simulink model "dbx_control_v0_02"  (R2015a)
settings: Solver=FixedStepDiscrete  SolverMode=SingleTasking  StartTime=0.0  StopTime=20  FixedStep=T_ctrl  RelTol=1e-3
values from neighbouring files (symbols this model uses):
  A_l_max_x = sqrt( (Max_Thrust*2/m)^2  -  (g*2/3)^2  )    [Run_DBX.m]    (also in simple_all.m = single(A_l_max_x))
  A_M = 2/sqrt(3)*L_M    [SetupComplete.m]    (also in simple_all.m = single(A_M))
  A_z_max = Max_Thrust*3/m    [Run_DBX.m]    (also in simple_all.m = single(A_z_max))
  CG = (m_OE*CG_OE + m_PL*CG_PL)/m    [SetupComplete.m]    (also in simple_all.m = single(CG))
  epsilon = 0.01    [Run_DBX.m]    (also in simple_all.m = single(epsilon))
  Flaps_ang_deg = 0    [FCS_fw_params.m]    (also in simple_all.m = single(Flaps_ang_deg))
  g = 9.81    [SetupComplete.m]    (also in simple_all.m = single(g))
  I_BAC = I_CG + m*[CG(3)^2,0,CG(1)*CG(3);0,CG(1)^2+CG(3)^2,0;CG(1)*CG(3),0,CG(1)^2]    [SetupComplete.m]    (also in simple_all.m = single(I_BAC))
  L_M = 1.20    (= 1.2)    [SetupComplete.m]    (also in simple_all.m = single(L_M))
  m = m_OE + m_PL    (= 14.5)    [SetupComplete.m]    (also in simple_all.m = single(m))
  Roll_pich_sens = single(Roll_pich_sens)    [simple_all.m]
  T_ctrl = 0.01    [Run_DBX.m]    (also in simple_all.m = double(T_ctrl))
  Throtle_sens = single(Throtle_sens)    [simple_all.m]
  v_i0 = sqrt( 1/3*m*g/(2*rho*pi*R^2)  )    [SetupComplete.m]    (also in simple_all.m = single(v_i0))
  Yaw_sens = single(Yaw_sens)    [simple_all.m]
undefined symbols (not defined in the file or in its folder): Hover_eta_23, Hover_throtle_1, Hover_throtle_23, Servo_calib
libraries: DBX_model x29, DBX_Control_lib x15, simulink x8, DBX_Control x3
(part 1 of 2)
settings Model: ExtModeTrigDuration=5000  TunableVars=Flaps_ang_deg,Roll_pich_sens,Throtle_sens,Yaw_sens,p_K_b,p_tau,phi_K_b,phi_f_i,phi_tau,psi_K_b,psi_f_i,psi_tau,q_K_b,q_tau,r_K_b,r_tau,theta_K_b,theta_f_i,theta_tau  TunableVarsStorageClass=Auto,Auto,Auto,Auto,Auto,Auto,Auto,Auto,Auto,Auto,Auto,Auto,Auto,Auto,Auto,Auto,Auto,Auto,Auto  TunableVarsTypeQualifier=,,,,,,,,,,,,,,,,,,  Creator=DavidTorres  LastModifiedBy=David
settings DataIOCC: LimitDataPoints=off  SaveOutput=off  SignalLogging=off  DSMLogging=off  VisualizeSimOutput=off  SaveTime=off
settings OptimizationCC: InlineParams=on  UseDivisionForNetSlopeComputation=on  UseSpecifiedMinMax=on  EfficientFloat2IntCast=on  OptimizeModelRefInitCode=on  MaxStackSize=64  SimCompilerOptimization=on
settings DebuggingCC: SaveWithParameterizedLinksMsg=none  IntegerOverflowMsg=error  StrictBusMsg=ErrorOnBusTreatedAsVector  IntegerSaturationMsg=error
settings HardwareCC: ProdLargestAtomicInteger=Long  ProdLargestAtomicFloat=Double  ProdIntDivRoundTo=Zero  ProdEndianess=LittleEndian  ProdHWDeviceType=Generic->32-bit x86 compatible  TargetLongLongMode=on  TargetIntDivRoundTo=Zero  TargetEndianess=LittleEndian  TargetHWDeviceType=MATLAB Host  ProdEqTarget=off
settings ModelReferenceCC: ModelReferenceNumInstancesAllowed=Single  ModelReferencePassRootInputsByReference=off
settings RTWCC: SystemTargetFile=ert.tlc  GenCodeOnly=on  TemplateMakefile=ert_default_tmf  Description=Embedded Coder  BuildConfiguration=Faster Runs
settings CodeAppCC: IgnoreCustomStorageClasses=off
settings ERTTargetCC: GenerateSampleERTMain=off  ParMdlRefBuildCompliant=on  CompOptLevelCompliant=on  ConcurrentExecutionCompliant=on  ERTFirstTimeCompliant=on  SupportNonFinite=off  SupportComplex=off  SupportContinuousTime=off  ModelStepFunctionPrototypeControlCompliant=on  CPPClassGenCompliant=on  InlinedParameterPlacement=Hierarchical  ERTCustomFileTemplate=example_file_process.tlc

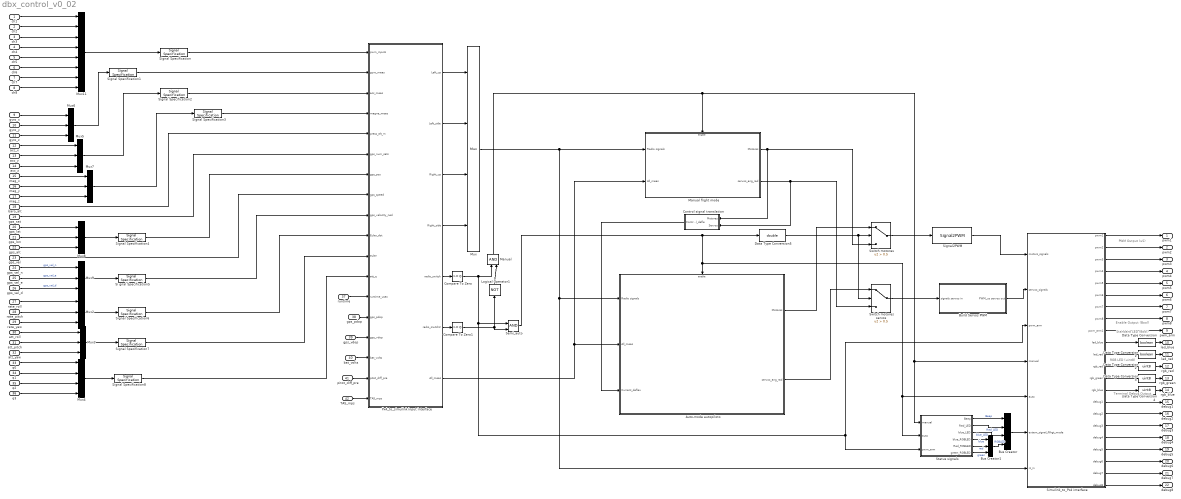
== system dbx_control_v0_02 ==
  note: Terminal Debug Output
  note: RGB LED (uint8)
  note: Standard LED (Bool)
  note: PWM Output (uS)
  note: Enable Output (Bool)
  ch1 : Inport  PortDimensions=[1,1]  SampleTime=T_ctrl
  ch2 : Inport  Port=2  PortDimensions=[1,1]  SampleTime=T_ctrl
  ch3 : Inport  Port=3  PortDimensions=[1,1]  SampleTime=T_ctrl
  ch4 : Inport  Port=4  PortDimensions=[1,1]  SampleTime=T_ctrl
  ch5 : Inport  Port=5  PortDimensions=[1,1]  SampleTime=T_ctrl
  ch6 : Inport  Port=6  PortDimensions=[1,1]  SampleTime=T_ctrl
  ch7 : Inport  Port=7  PortDimensions=[1,1]  SampleTime=T_ctrl
  ch8 : Inport  Port=8  PortDimensions=[1,1]  SampleTime=T_ctrl
  gyro_x : Inport  Port=9  PortDimensions=[1,1]  SampleTime=T_ctrl
  gyro_y : Inport  Port=10  PortDimensions=[1,1]  SampleTime=T_ctrl
  gyro_z : Inport  Port=11  PortDimensions=[1,1]  SampleTime=T_ctrl
  acc_x : Inport  Port=12  PortDimensions=[1,1]  SampleTime=T_ctrl
  acc_y : Inport  Port=13  PortDimensions=[1,1]  SampleTime=T_ctrl
  acc_z : Inport  Port=14  PortDimensions=[1,1]  SampleTime=T_ctrl
  mag_x : Inport  Port=15  PortDimensions=[1,1]  SampleTime=T_ctrl
  mag_y : Inport  Port=16  PortDimensions=[1,1]  SampleTime=T_ctrl
  mag_z : Inport  Port=17  PortDimensions=[1,1]  SampleTime=T_ctrl
  baro_alt : Inport  Port=18  PortDimensions=[1,1]  SampleTime=T_ctrl
  gps_sat : Inport  Port=19  PortDimensions=[1,1]  SampleTime=T_ctrl
  gps_lat : Inport  Port=20  PortDimensions=[1,1]  SampleTime=T_ctrl
  gps_lon : Inport  Port=21  PortDimensions=[1,1]  SampleTime=T_ctrl
  gps_alt : Inport  Port=22  PortDimensions=[1,1]  SampleTime=T_ctrl
  gps_vel : Inport  Port=23  PortDimensions=[1,1]  SampleTime=T_ctrl
  gps_vel_n : Inport  Port=24  PortDimensions=[1,1]  SampleTime=T_ctrl
  gps_vel_e : Inport  Port=25  PortDimensions=[1,1]  SampleTime=T_ctrl
  gps_vel_d : Inport  Port=26  PortDimensions=[1,1]  SampleTime=T_ctrl
  rate_roll : Inport  Port=27  PortDimensions=[1,1]  SampleTime=T_ctrl
  rate_pitch : Inport  Port=28  PortDimensions=[1,1]  SampleTime=T_ctrl
  rate_yaw : Inport  Port=29  PortDimensions=[1,1]  SampleTime=T_ctrl
  att_roll : Inport  Port=30  PortDimensions=[1,1]  SampleTime=T_ctrl
  att_pitch : Inport  Port=31  PortDimensions=[1,1]  SampleTime=T_ctrl
  att_yaw : Inport  Port=32  PortDimensions=[1,1]  SampleTime=T_ctrl
  q0 : Inport  Port=33  PortDimensions=[1,1]  SampleTime=T_ctrl
  q1 : Inport  Port=34  PortDimensions=[1,1]  SampleTime=T_ctrl
  q2 : Inport  Port=35  PortDimensions=[1,1]  SampleTime=T_ctrl
  q3 : Inport  Port=36  PortDimensions=[1,1]  SampleTime=T_ctrl
  runtime : Inport  Port=37  PortDimensions=[1,1]  SampleTime=T_ctrl
  gps_pdop : Inport  Port=38  PortDimensions=[1,1]  SampleTime=T_ctrl
  gps_vdop : Inport  Port=39  PortDimensions=[1,1]  SampleTime=T_ctrl
  bat_volts : Inport  Port=40  PortDimensions=[1,1]  SampleTime=T_ctrl
  pitot_diff_pre : Inport  Port=41  SampleTime=T_ctrl
  TAS_mps : Inport  Port=42  SampleTime=T_ctrl
  Auto-mode autopiloto : Subsystem  TreatAsAtomicUnit=on
  Build Servos PWM : Subsystem  TreatAsAtomicUnit=on
  Bus Creator : BusCreator
  Bus Creator1 : BusCreator  Inputs=3
  Compare To Zero : simulink/Logic and Bit Operations/Compare To Zero  relop=>=  OutDataTypeStr=boolean
  Compare To Zero1 : simulink/Logic and Bit Operations/Compare To Zero  relop=>=  OutDataTypeStr=boolean
  Control signal translation : Subsystem  TreatAsAtomicUnit=on
  Data Type Conversion : DataTypeConversion  OutDataTypeStr=boolean
  Data Type Conversion1 : DataTypeConversion  OutDataTypeStr=boolean
  Data Type Conversion2 : DataTypeConversion  OutDataTypeStr=uint8
  Data Type Conversion3 : DataTypeConversion  OutDataTypeStr=uint8
  Data Type Conversion4 : DataTypeConversion  OutDataTypeStr=uint8
  Data Type Conversion5 : DataTypeConversion  OutDataTypeStr=double
  Logical Operator1 : Logic  Operator=NOT  IconShape=distinctive  AllPortsSameDT=off  OutDataTypeStr=boolean
  Manual : Logic  IconShape=distinctive  AllPortsSameDT=off  OutDataTypeStr=boolean
  Manual flight mode : Subsystem  TreatAsAtomicUnit=on
  Mux : Mux
  Mux11 : Mux  Inputs=8
  Mux{2..3,5..9} (7 alike) : Mux  Inputs=3
  Mux4 : Mux
  Px4_to_simulink input interface : Subsystem
  Semi_auto : Logic  IconShape=distinctive  AllPortsSameDT=off  OutDataTypeStr=boolean
  Si gnal Specification5 : SignalSpecification  Dimensions=[3,1]
  Signal Specification : SignalSpecification  Dimensions=[8,1]
  Signal Specification{1..4,6..7} (6 alike) : SignalSpecification  Dimensions=[3,1]
  Signal Specification8 : SignalSpecification  Dimensions=[4,1]
  Signal2PWM : DBX_model/Signal2PWM  b=1  d=0  a=1900  c=1100
  Simulink_to_Px4 interface : Subsystem
  Status signals : Subsystem  TreatAsAtomicUnit=on
  Switch motores : Switch  Criteria=u2 > Threshold  Threshold=0.5
  Switch motores servos : Switch  Criteria=u2 > Threshold  Threshold=0.5
  pwm1 : Outport  PortDimensions=[1,1]
  pwm2 : Outport  Port=2  PortDimensions=[1,1]
  pwm3 : Outport  Port=3  PortDimensions=[1,1]
  pwm4 : Outport  Port=4  PortDimensions=[1,1]
  pwm5 : Outport  Port=5  PortDimensions=[1,1]
  pwm6 : Outport  Port=6  PortDimensions=[1,1]
  pwm7 : Outport  Port=7  PortDimensions=[1,1]
  pwm8 : Outport  Port=8  PortDimensions=[1,1]
  pwm_arm : Outport  Port=9  PortDimensions=[1,1]
  led_blue : Outport  Port=10  OutDataTypeStr=boolean  PortDimensions=[1,1]
  led_red : Outport  Port=11  OutDataTypeStr=boolean  PortDimensions=[1,1]
  rgb_red : Outport  Port=12  OutDataTypeStr=uint8  PortDimensions=[1,1]
  rgb_green : Outport  Port=13  OutDataTypeStr=uint8  PortDimensions=[1,1]
  rgb_blue : Outport  Port=14  OutDataTypeStr=uint8  PortDimensions=[1,1]
  debug1 : Outport  Port=15  PortDimensions=[1,1]
  debug2 : Outport  Port=16  PortDimensions=[1,1]
  debug3 : Outport  Port=17  PortDimensions=[1,1]
  debug4 : Outport  Port=18  PortDimensions=[1,1]
  debug5 : Outport  Port=19  PortDimensions=[1,1]
  debug6 : Outport  Port=20  PortDimensions=[1,1]
  debug7 : Outport  Port=21  PortDimensions=[1,1]
  debug8 : Outport  Port=22  PortDimensions=[1,1]
  wires:
  Switch motores/1 -> Signal2PWM/1
  Switch motores servos/1 -> Build Servos PWM/1(signals servos in)
  Status signals/1(Beep) -> Bus Creator/1  "Beep"
  Status signals/2(Red_LED) -> Bus Creator/2  "Red_LED"
  Status signals/3(blue_LED) -> Bus Creator/3  "blue_LED"
  Status signals/4(blue_RGBLED) -> Bus Creator1/1  "blue"
  Status signals/5(Red_RGBLED) -> Bus Creator1/2  "red"
  Status signals/6(green_RGBLED) -> Bus Creator1/3  "green"
  Bus Creator1/1 -> Bus Creator/4  "RGBLED"
  Simulink_to_Px4 interface/1(pwm1) -> pwm1/1
  Simulink_to_Px4 interface/2(pwm2) -> pwm2/1
  Simulink_to_Px4 interface/3(pwm3) -> pwm3/1
  Simulink_to_Px4 interface/4(pwm4) -> pwm4/1
  Simulink_to_Px4 interface/5(pwm5) -> pwm5/1
  Simulink_to_Px4 interface/6(pwm6) -> pwm6/1
  Simulink_to_Px4 interface/7(pwm7) -> pwm7/1
  Simulink_to_Px4 interface/8(pwm8) -> pwm8/1
  Simulink_to_Px4 interface/10(led_blue) -> Data Type Conversion/1
  Simulink_to_Px4 interface/11(led_red) -> Data Type Conversion1/1
  Simulink_to_Px4 interface/15(debug1) -> debug1/1
  Simulink_to_Px4 interface/17(debug3) -> debug3/1
  Simulink_to_Px4 interface/18(debug4) -> debug4/1
  Simulink_to_Px4 interface/9(pwm_arm1) -> pwm_arm/1
  Simulink_to_Px4 interface/12(rgb_red) -> Data Type Conversion2/1
  Simulink_to_Px4 interface/13(rgb_green) -> Data Type Conversion3/1
  Simulink_to_Px4 interface/14(rgb_blue) -> Data Type Conversion4/1
  Simulink_to_Px4 interface/20(debug6) -> debug6/1
  Simulink_to_Px4 interface/21(debug7) -> debug7/1
  Simulink_to_Px4 interface/22(debug8) -> debug8/1
  Simulink_to_Px4 interface/19(debug5) -> debug5/1
  Data Type Conversion/1 -> led_blue/1
  Data Type Conversion1/1 -> led_red/1
  Data Type Conversion2/1 -> rgb_red/1
  Data Type Conversion3/1 -> rgb_green/1
  Data Type Conversion4/1 -> rgb_blue/1
  Simulink_to_Px4 interface/16(debug2) -> debug2/1
  Signal2PWM/1 -> Simulink_to_Px4 interface/1(motors_signals)
  Build Servos PWM/1(PWM_us servos out) -> Simulink_to_Px4 interface/2(servos_signals)
  Bus Creator/1 -> Simulink_to_Px4 interface/6(extern_signal_flihgt_mode)
  baro_alt/1 -> Px4_to_simulink input interface/5(press_alt_m)
  gyro_z/1 -> Mux6/3
  gyro_y/1 -> Mux6/2
  gyro_x/1 -> Mux6/1
  acc_z/1 -> Mux5/3
  acc_y/1 -> Mux5/2
  acc_x/1 -> Mux5/1
  mag_x/1 -> Mux7/1
  mag_y/1 -> Mux7/2
  mag_z/1 -> Mux7/3
  ch1/1 -> Mux11/1
  ch2/1 -> Mux11/2
  ch3/1 -> Mux11/3
  ch4/1 -> Mux11/4
  ch5/1 -> Mux11/5
  ch6/1 -> Mux11/6
  runtime/1 -> Px4_to_simulink input interface/13(runtime_usec)
  ch7/1 -> Mux11/7
  ch8/1 -> Mux11/8
  att_roll/1 -> Mux3/1
  att_pitch/1 -> Mux3/2
  att_yaw/1 -> Mux3/3
  q0/1 -> Mux4/1
  q1/1 -> Mux4/2
  q2/1 -> Mux4/3
  q3/1 -> Mux4/4
  rate_roll/1 -> Mux2/1
  rate_pitch/1 -> Mux2/2
  rate_yaw/1 -> Mux2/3
  gps_vel_n/1 -> Mux9/1  "gps_vel_n"
  gps_vel_e/1 -> Mux9/2  "gps_vel_e"
  gps_vel_d/1 -> Mux9/3  "gps_vel_d"
  gps_lat/1 -> Mux8/1
  gps_lon/1 -> Mux8/2
  gps_alt/1 -> Mux8/3
  gps_vel/1 -> Px4_to_simulink input interface/8(gps_speed)
  gps_sat/1 -> Px4_to_simulink input interface/6(gps_num_sats)
  Mux2/1 -> Signal Specification6/1
  Mux3/1 -> Signal Specification7/1
  Mux4/1 -> Signal Specification8/1
  Mux5/1 -> Signal Specification2/1
  Mux6/1 -> Signal Specification1/1
  Mux8/1 -> Signal Specification4/1
  Mux7/1 -> Signal Specification3/1
  Mux11/1 -> Signal Specification/1
  Mux9/1 -> Si gnal Specification5/1
  gps_pdop/1 -> Px4_to_simulink input interface/14(gps_pdop)
  gps_vdop/1 -> Px4_to_simulink input interface/15(gps_vdop)
  bat_volts/1 -> Px4_to_simulink input interface/16(bat_volts)
  Signal Specification/1 -> Px4_to_simulink input interface/1(pwm_inputs)
  Signal Specification1/1 -> Px4_to_simulink input interface/2(gyro_meas)
  Signal Specification2/1 -> Px4_to_simulink input interface/3(acc_meas)
  Signal Specification3/1 -> Px4_to_simulink input interface/4(magne_meas)
  Signal Specification4/1 -> Px4_to_simulink input interface/7(gps_pos)
  Si gnal Specification5/1 -> Px4_to_simulink input interface/9(gps_velocity_ned)
  Signal Specification6/1 -> Px4_to_simulink input interface/10(Euler_dot)
  Signal Specification7/1 -> Px4_to_simulink input interface/11(euler)
  Signal Specification8/1 -> Px4_to_simulink input interface/12(att_q)
  pitot_diff_pre/1 -> Px4_to_simulink input interface/17(pitot_diff_pre)
  Px4_to_simulink input interface/5(radio_switch) -> Compare To Zero/1
  Px4_to_simulink input interface/6(radio_siwtch2) -> Compare To Zero1/1
  Compare To Zero/1 -> Semi_auto/1, Simulink_to_Px4 interface/3(pwm_arm), Status signals/3(pwm_arm), Manual/1
  Compare To Zero1/1 -> Logical Operator1/1, Semi_auto/2
  Manual/1 -> Simulink_to_Px4 interface/4(manual), Status signals/1(manual), Manual flight mode/Enable
  Manual flight mode/2(servos_ang_rad) -> Control signal translation/2(Servos), Switch motores servos/3
  Auto-mode autopiloto/1(Motores) -> Switch motores/1
  Auto-mode autopiloto/2(servos_ang_rad) -> Switch motores servos/1
  Semi_auto/1 -> Data Type Conversion5/1, Simulink_to_Px4 interface/5(auto), Status signals/2(auto), Auto-mode autopiloto/Enable
  Data Type Conversion5/1 -> Switch motores servos/2, Switch motores/2
  Px4_to_simulink input interface/4(Right_side) -> Mux/4
  Px4_to_simulink input interface/3(Right_up) -> Mux/3
  Px4_to_simulink input interface/2(Left_side) -> Mux/2
  Px4_to_simulink input interface/1(Left_up) -> Mux/1
  Px4_to_simulink input interface/7(All_meas) -> Manual flight mode/2(All_meas), Auto-mode autopiloto/2(All_meas)
  Mux/1 -> Manual flight mode/1(Radio signals), Simulink_to_Px4 interface/7(rc_in), Auto-mode autopiloto/1(Radio signals)
  TAS_mps/1 -> Px4_to_simulink input interface/18(TAS_mps)
  Logical Operator1/1 -> Manual/2
  Manual flight mode/1(Motores) -> Switch motores/3, Control signal translation/1(Motores)
  Control signal translation/1(Control_defle) -> Auto-mode autopiloto/3(Current_deflex)

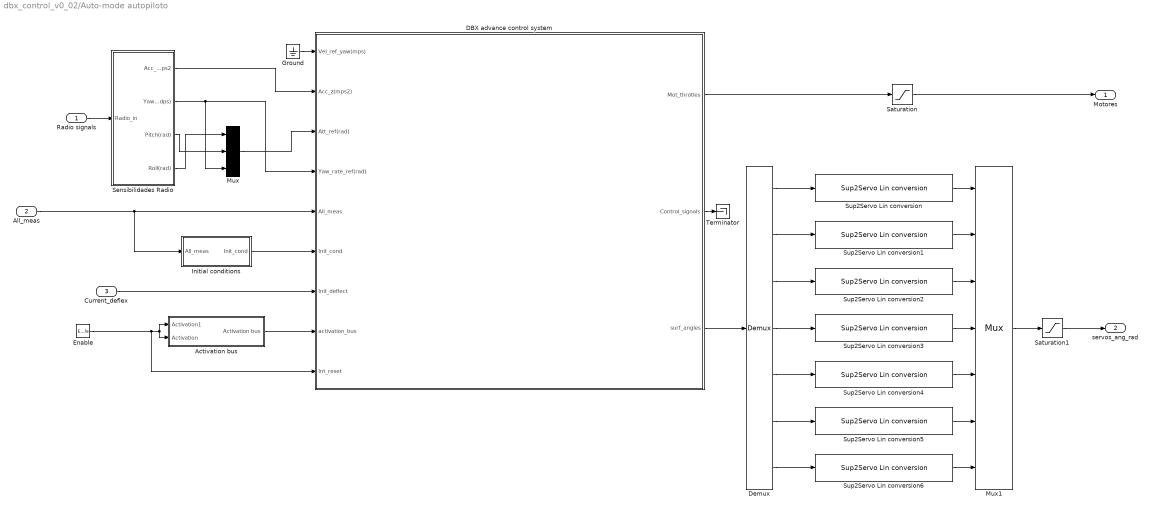
== system dbx_control_v0_02/Auto-mode autopiloto ==
  Radio signals : Inport
  All_meas : Inport  Port=2
  Current_deflex : Inport  Port=3
  Enable : EnablePort  ShowOutputPort=on
  Activation bus : Subsystem  TreatAsAtomicUnit=on
  DBX advance control system : Subsystem
  Demux : Demux  Outputs=7
  "Ground " : Ground
  Initial conditions : Subsystem  TreatAsAtomicUnit=on
  Mux : Mux  Inputs=3
  Mux1 : Mux  Inputs=7
  Saturation : Saturate  UpperLimit=1  LowerLimit=0
  Saturation1 : Saturate  UpperLimit=deg2rad(90)  LowerLimit=-deg2rad(90)
  Sensibilidades Radio : Subsystem  TreatAsAtomicUnit=on
  Sup2Servo Lin conversion : DBX_model/Sup2Servo Lin conversion  Gain=Servo_calib.Servo1.Pendiente_Sup_Servo  Bias=Servo_calib.Servo1.Sup_rad_0
  Sup2Servo Lin conversion1 : DBX_model/Sup2Servo Lin conversion  Gain=Servo_calib.Servo2.Pendiente_Sup_Servo  Bias=Servo_calib.Servo2.Sup_rad_0
  Sup2Servo Lin conversion2 : DBX_model/Sup2Servo Lin conversion  Gain=Servo_calib.Servo3.Pendiente_Sup_Servo  Bias=Servo_calib.Servo3.Sup_rad_0
  Sup2Servo Lin conversion3 : DBX_model/Sup2Servo Lin conversion  Gain=Servo_calib.Servo4.Pendiente_Sup_Servo  Bias=Servo_calib.Servo4.Sup_rad_0
  Sup2Servo Lin conversion4 : DBX_model/Sup2Servo Lin conversion  Gain=Servo_calib.Servo5.Pendiente_Sup_Servo  Bias=Servo_calib.Servo5.Sup_rad_0
  Sup2Servo Lin conversion5 : DBX_model/Sup2Servo Lin conversion  Gain=Servo_calib.Servo6.Pendiente_Sup_Servo  Bias=Servo_calib.Servo6.Sup_rad_0
  Sup2Servo Lin conversion6 : DBX_model/Sup2Servo Lin conversion  Gain=Servo_calib.Servo7.Pendiente_Sup_Servo  Bias=Servo_calib.Servo7.Sup_rad_0
  Terminator : Terminator
  Motores : Outport
  servos_ang_rad : Outport  Port=2
  wires:
  DBX advance control system/1(Mot_throtles) -> Saturation/1
  Saturation/1 -> Motores/1
  Mux1/1 -> Saturation1/1
  Saturation1/1 -> servos_ang_rad/1
  Sup2Servo Lin conversion/1 -> Mux1/1
  Sup2Servo Lin conversion1/1 -> Mux1/2
  Sup2Servo Lin conversion2/1 -> Mux1/3
  Sup2Servo Lin conversion3/1 -> Mux1/4
  Sup2Servo Lin conversion4/1 -> Mux1/5
  Sup2Servo Lin conversion5/1 -> Mux1/6
  Sup2Servo Lin conversion6/1 -> Mux1/7
  All_meas/1 -> Initial conditions/1(All_meas), DBX advance control system/5(All_meas)
  DBX advance control system/3(surf_angles) -> Demux/1
  Demux/1 -> Sup2Servo Lin conversion/1
  Demux/2 -> Sup2Servo Lin conversion1/1
  Demux/3 -> Sup2Servo Lin conversion2/1
  Demux/4 -> Sup2Servo Lin conversion3/1
  Demux/5 -> Sup2Servo Lin conversion4/1
  Demux/6 -> Sup2Servo Lin conversion5/1
  Demux/7 -> Sup2Servo Lin conversion6/1
  Radio signals/1 -> Sensibilidades Radio/1(Radio_in)
  Sensibilidades Radio/1(Acc_z_mps2) -> DBX advance control system/2(Acc_z(mps2))
  Mux/1 -> DBX advance control system/3(Att_ref(rad))
  "Ground "/1 -> DBX advance control system/1(Vel_ref_yaw(mps))
  Sensibilidades Radio/2(Yaw(radps)) -> Mux/3, DBX advance control system/4(Yaw_rate_ref(rad))
  Sensibilidades Radio/4(Roll(rad)) -> Mux/1
  Sensibilidades Radio/3(Pitch(rad)) -> Mux/2
  Activation bus/1(Activation bus) -> DBX advance control system/8(activation_bus)
  Enable/1 -> DBX advance control system/9(Int_reset), Activation bus/2(Activation), Activation bus/1(Activation1)
  Initial conditions/1(Init_cond) -> DBX advance control system/6(Init_cond)
  Current_deflex/1 -> DBX advance control system/7(Init_deflect)
  DBX advance control system/2(Control_signals) -> Terminator/1

== system dbx_control_v0_02/Build Servos PWM ==
  note: Estos 4 ultimos significa que
      | los ejes de los servos deben
      | apuntar el la direccion +y
  note: Control input
      | Rango
      | Direccion rot/Dir servos
      | Rango del servo
      |
      | eta_1 (rad) (Pan arm 1)
      | -90,90
      | -1
      | 180
      |
      | eta_2 (rad) (Pan arm 2
      | -90,90
      | -1
      | 180
      |
      | eta_3 (rad) (Pan arm 3)
      | -90,90
      | 1
      | 180
      |
      | Rudervator Left (rad)
      | -90,90
      | 1
      | 180
      |
      | Rudervator Right (rad)
      | -90,90
      | 1
      | 180
      |
      | Aileron Left (rad)
      | -90,90
      | 1
      | 180
      |
      | Aielron Right (rad)
      | -90,90
      | 1
      | 180
  signals servos in : Inport
  Demux : Demux  Outputs=7
  Mux : Mux  Inputs=7
  Signal2PWM{,1..6} (7 alike) : DBX_model/Signal2PWM  b=deg2rad(90)  d=-deg2rad(90)  a=1900  c=1100
  PWM_us servos out : Outport
  wires:
  Mux/1 -> PWM_us servos out/1
  signals servos in/1 -> Demux/1
  Demux/6 -> Signal2PWM5/1
  Demux/5 -> Signal2PWM4/1
  Demux/4 -> Signal2PWM3/1
  Demux/3 -> Signal2PWM2/1
  Demux/2 -> Signal2PWM1/1
  Demux/1 -> Signal2PWM/1
  Signal2PWM/1 -> Mux/1
  Signal2PWM1/1 -> Mux/2
  Signal2PWM3/1 -> Mux/4
  Signal2PWM4/1 -> Mux/5
  Signal2PWM2/1 -> Mux/3
  Signal2PWM5/1 -> Mux/6
  Demux/7 -> Signal2PWM6/1
  Signal2PWM6/1 -> Mux/7

== system dbx_control_v0_02/Control signal translation ==
  Motores : Inport
  Servos : Inport  Port=2
  Demux : Demux  Outputs=3
  Ground{,1..4} (5 alike) : Ground
  Mux1 : Mux  Inputs=9
  Selector : Selector  InputPortWidth=7  Indices=3
  Servo2Sup Lin conversion : DBX_model/Servo2Sup Lin conversion  Gain=Servo_calib.Servo3.Pendiente_Sup_Servo  Bias=Servo_calib.Servo3.Sup_rad_0
  Control_defle : Outport
  wires:
  Mux1/1 -> Control_defle/1
  Demux/1 -> Mux1/1
  Servos/1 -> Selector/1
  Demux/2 -> Mux1/3
  Demux/3 -> Mux1/5
  Ground/1 -> Mux1/2
  Ground1/1 -> Mux1/4
  Ground2/1 -> Mux1/7
  Ground3/1 -> Mux1/8
  Ground4/1 -> Mux1/9
  Servo2Sup Lin conversion/1 -> Mux1/6
  Motores/1 -> Demux/1
  Selector/1 -> Servo2Sup Lin conversion/1

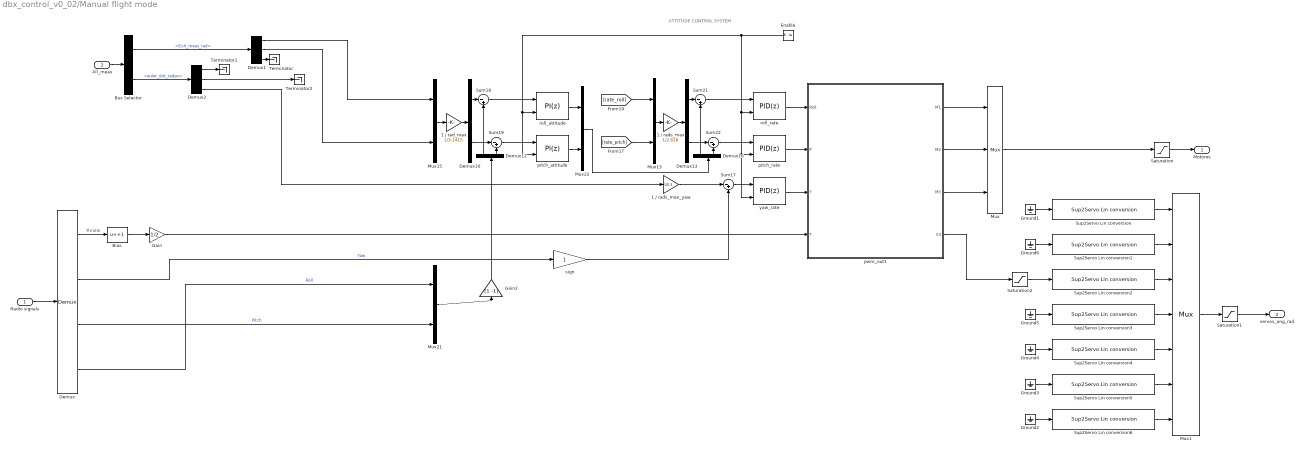
== system dbx_control_v0_02/Manual flight mode ==
  note: ATTITUDE CONTROL SYSTEM
  Radio signals : Inport
  All_meas : Inport  Port=2
  Enable : EnablePort  ShowOutputPort=on
  1 / rad_max : Gain  Gain=1/3.1415
  1 / rads_max : Gain  Gain=1/2.618
  1 / rads_max_yaw : Gain  Gain=1/5.3
  Bias : Bias  Bias=+1
  Bus Selector : BusSelector  OutputSignals=Meas.Eulr_meas_rad,Meas.euler_dot_radps
  Demux : Demux
  Demux1 : Demux  Outputs=3
  Demux{10,12..13,16} (4 alike) : Demux  Outputs=2
  Demux2 : Demux  Outputs=3
  Gain : Gain  Gain=1/2
  Gain2 : Gain  Gain=[1 -1]
  Ground{1..6} (6 alike) : Ground
  Mux : Mux  Inputs=3
  Mux1 : Mux  Inputs=7
  Mux{13,15,21..22} (4 alike) : Mux  Inputs=2
  Saturation : Saturate  UpperLimit=1  LowerLimit=0
  Saturation1 : Saturate  UpperLimit=deg2rad(90)  LowerLimit=-deg2rad(90)
  Saturation2 : Saturate  UpperLimit=deg2rad(20)  LowerLimit=-deg2rad(20)
  Sum{17..19,21..22} (5 alike) : Sum  Inputs=|-+
  Sup2Servo Lin conversion : DBX_model/Sup2Servo Lin conversion  Gain=Servo_calib.Servo1.Pendiente_Sup_Servo  Bias=Servo_calib.Servo1.Sup_rad_0
  Sup2Servo Lin conversion1 : DBX_model/Sup2Servo Lin conversion  Gain=Servo_calib.Servo2.Pendiente_Sup_Servo  Bias=Servo_calib.Servo2.Sup_rad_0
  Sup2Servo Lin conversion2 : DBX_model/Sup2Servo Lin conversion  Gain=Servo_calib.Servo3.Pendiente_Sup_Servo  Bias=Servo_calib.Servo3.Sup_rad_0
  Sup2Servo Lin conversion3 : DBX_model/Sup2Servo Lin conversion  Gain=Servo_calib.Servo4.Pendiente_Sup_Servo  Bias=Servo_calib.Servo4.Sup_rad_0
  Sup2Servo Lin conversion4 : DBX_model/Sup2Servo Lin conversion  Gain=Servo_calib.Servo5.Pendiente_Sup_Servo  Bias=Servo_calib.Servo5.Sup_rad_0
  Sup2Servo Lin conversion5 : DBX_model/Sup2Servo Lin conversion  Gain=Servo_calib.Servo6.Pendiente_Sup_Servo  Bias=Servo_calib.Servo6.Sup_rad_0
  Sup2Servo Lin conversion6 : DBX_model/Sup2Servo Lin conversion  Gain=Servo_calib.Servo7.Pendiente_Sup_Servo  Bias=Servo_calib.Servo7.Sup_rad_0
  Terminator : Terminator
  Terminator1 : Terminator
  Terminator2 : Terminator
  pitch_attitude : simulink/Continuous/PID Controller  Controller=PI  TimeDomain=Discrete-time  SampleTime=-1  IntegratorMethod=Forward Euler  FilterMethod=Forward Euler  Form=Parallel  UseFilter=on  ControllerParametersSource=internal  P=0.4  I=0.1  D=0  N=100  InitialConditionSource=internal  InitialConditionForIntegrator=0  InitialConditionForFilter=0  ExternalReset=either  LimitOutput=on  UpperSaturationLimit=1  LowerSaturationLimit=-1  LinearizeAsGain=on  AntiWindupMode=none  Kb=1  TrackingMode=off  Kt=1  PParamMin=[]  PParamMax=[]  IParamMin=[]  IParamMax=[]  DParamMin=[]  DParamMax=[]  NParamMin=[]  NParamMax=[]  KbParamMin=[]  KbParamMax=[]  KtParamMin=[]  KtParamMax=[]  POutMin=[]  POutMax=[]  IOutMin=[]  IOutMax=[]  DOutMin=[]  DOutMax=[]  NOutMin=[]  NOutMax=[]  KbOutMin=[]  KbOutMax=[]  KtOutMin=[]  KtOutMax=[]  IntegratorOutMin=[]  IntegratorOutMax=[]  FilterOutMin=[]  FilterOutMax=[]  SumOutMin=[]  SumOutMax=[]  SumI1OutMin=[]  SumI1OutMax=[]  SumI2OutMin=[]  SumI2OutMax=[]  SumI3OutMin=[]  SumI3OutMax=[]  SumDOutMin=[]  SumDOutMax=[]  SaturationOutMin=[]  SaturationOutMax=[]  IntegratorContinuousStateAttributes=''  IntegratorStateMustResolveToSignalObject=off  IntegratorRTWStateStorageClass=Auto  FilterContinuousStateAttributes=''  FilterStateMustResolveToSignalObject=off  FilterRTWStateStorageClass=Auto  DifferentiatorICPrevScaledInput=0  DifferentiatorOutMin=[]  DifferentiatorOutMax=[]
  pitch_rate : simulink/Continuous/PID Controller  Controller=PID  TimeDomain=Discrete-time  SampleTime=-1  IntegratorMethod=Forward Euler  FilterMethod=Forward Euler  Form=Parallel  UseFilter=on  ControllerParametersSource=internal  P=0.1  I=0  D=0  N=100  InitialConditionSource=internal  InitialConditionForIntegrator=0  InitialConditionForFilter=0  ExternalReset=either  LimitOutput=on  UpperSaturationLimit=1  LowerSaturationLimit=-1  LinearizeAsGain=on  AntiWindupMode=none  Kb=1  TrackingMode=off  Kt=1  PParamMin=[]  PParamMax=[]  IParamMin=[]  IParamMax=[]  DParamMin=[]  DParamMax=[]  NParamMin=[]  NParamMax=[]  KbParamMin=[]  KbParamMax=[]  KtParamMin=[]  KtParamMax=[]  POutMin=[]  POutMax=[]  IOutMin=[]  IOutMax=[]  DOutMin=[]  DOutMax=[]  NOutMin=[]  NOutMax=[]  KbOutMin=[]  KbOutMax=[]  KtOutMin=[]  KtOutMax=[]  IntegratorOutMin=[]  IntegratorOutMax=[]  FilterOutMin=[]  FilterOutMax=[]  SumOutMin=[]  SumOutMax=[]  SumI1OutMin=[]  SumI1OutMax=[]  SumI2OutMin=[]  SumI2OutMax=[]  SumI3OutMin=[]  SumI3OutMax=[]  SumDOutMin=[]  SumDOutMax=[]  SaturationOutMin=[]  SaturationOutMax=[]  IntegratorContinuousStateAttributes=''  IntegratorStateMustResolveToSignalObject=off  IntegratorRTWStateStorageClass=Auto  FilterContinuousStateAttributes=''  FilterStateMustResolveToSignalObject=off  FilterRTWStateStorageClass=Auto  DifferentiatorICPrevScaledInput=0  DifferentiatorOutMin=[]  DifferentiatorOutMax=[]
  pwm_out1 : MATLAB Function  TreatAsAtomicUnit=on  SystemSampleTime=T_ctrl
  roll_attitude : simulink/Continuous/PID Controller  Controller=PI  TimeDomain=Discrete-time  SampleTime=-1  IntegratorMethod=Forward Euler  FilterMethod=Forward Euler  Form=Parallel  UseFilter=on  ControllerParametersSource=internal  P=0.4  I=0.1  D=0  N=100  InitialConditionSource=internal  InitialConditionForIntegrator=0  InitialConditionForFilter=0  ExternalReset=either  LimitOutput=on  UpperSaturationLimit=1  LowerSaturationLimit=-1  LinearizeAsGain=on  AntiWindupMode=none  Kb=1  TrackingMode=off  Kt=1  PParamMin=[]  PParamMax=[]  IParamMin=[]  IParamMax=[]  DParamMin=[]  DParamMax=[]  NParamMin=[]  NParamMax=[]  KbParamMin=[]  KbParamMax=[]  KtParamMin=[]  KtParamMax=[]  POutMin=[]  POutMax=[]  IOutMin=[]  IOutMax=[]  DOutMin=[]  DOutMax=[]  NOutMin=[]  NOutMax=[]  KbOutMin=[]  KbOutMax=[]  KtOutMin=[]  KtOutMax=[]  IntegratorOutMin=[]  IntegratorOutMax=[]  FilterOutMin=[]  FilterOutMax=[]  SumOutMin=[]  SumOutMax=[]  SumI1OutMin=[]  SumI1OutMax=[]  SumI2OutMin=[]  SumI2OutMax=[]  SumI3OutMin=[]  SumI3OutMax=[]  SumDOutMin=[]  SumDOutMax=[]  SaturationOutMin=[]  SaturationOutMax=[]  IntegratorContinuousStateAttributes=''  IntegratorStateMustResolveToSignalObject=off  IntegratorRTWStateStorageClass=Auto  FilterContinuousStateAttributes=''  FilterStateMustResolveToSignalObject=off  FilterRTWStateStorageClass=Auto  DifferentiatorICPrevScaledInput=0  DifferentiatorOutMin=[]  DifferentiatorOutMax=[]
  roll_rate : simulink/Continuous/PID Controller  Controller=PID  TimeDomain=Discrete-time  SampleTime=-1  IntegratorMethod=Forward Euler  FilterMethod=Forward Euler  Form=Parallel  UseFilter=on  ControllerParametersSource=internal  P=0.1  I=0  D=0  N=100  InitialConditionSource=internal  InitialConditionForIntegrator=0  InitialConditionForFilter=0  ExternalReset=either  LimitOutput=on  UpperSaturationLimit=1  LowerSaturationLimit=-1  LinearizeAsGain=on  AntiWindupMode=none  Kb=1  TrackingMode=off  Kt=1  PParamMin=[]  PParamMax=[]  IParamMin=[]  IParamMax=[]  DParamMin=[]  DParamMax=[]  NParamMin=[]  NParamMax=[]  KbParamMin=[]  KbParamMax=[]  KtParamMin=[]  KtParamMax=[]  POutMin=[]  POutMax=[]  IOutMin=[]  IOutMax=[]  DOutMin=[]  DOutMax=[]  NOutMin=[]  NOutMax=[]  KbOutMin=[]  KbOutMax=[]  KtOutMin=[]  KtOutMax=[]  IntegratorOutMin=[]  IntegratorOutMax=[]  FilterOutMin=[]  FilterOutMax=[]  SumOutMin=[]  SumOutMax=[]  SumI1OutMin=[]  SumI1OutMax=[]  SumI2OutMin=[]  SumI2OutMax=[]  SumI3OutMin=[]  SumI3OutMax=[]  SumDOutMin=[]  SumDOutMax=[]  SaturationOutMin=[]  SaturationOutMax=[]  IntegratorContinuousStateAttributes=''  IntegratorStateMustResolveToSignalObject=off  IntegratorRTWStateStorageClass=Auto  FilterContinuousStateAttributes=''  FilterStateMustResolveToSignalObject=off  FilterRTWStateStorageClass=Auto  DifferentiatorICPrevScaledInput=0  DifferentiatorOutMin=[]  DifferentiatorOutMax=[]
  sign : Gain
  yaw_rate : simulink/Continuous/PID Controller  Controller=PID  TimeDomain=Discrete-time  SampleTime=-1  IntegratorMethod=Forward Euler  FilterMethod=Forward Euler  Form=Parallel  UseFilter=on  ControllerParametersSource=internal  P=2  I=0.2  D=0  N=100  InitialConditionSource=internal  InitialConditionForIntegrator=0  InitialConditionForFilter=0  ExternalReset=either  LimitOutput=on  UpperSaturationLimit=1  LowerSaturationLimit=-1  LinearizeAsGain=on  AntiWindupMode=none  Kb=1  TrackingMode=off  Kt=1  PParamMin=[]  PParamMax=[]  IParamMin=[]  IParamMax=[]  DParamMin=[]  DParamMax=[]  NParamMin=[]  NParamMax=[]  KbParamMin=[]  KbParamMax=[]  KtParamMin=[]  KtParamMax=[]  POutMin=[]  POutMax=[]  IOutMin=[]  IOutMax=[]  DOutMin=[]  DOutMax=[]  NOutMin=[]  NOutMax=[]  KbOutMin=[]  KbOutMax=[]  KtOutMin=[]  KtOutMax=[]  IntegratorOutMin=[]  IntegratorOutMax=[]  FilterOutMin=[]  FilterOutMax=[]  SumOutMin=[]  SumOutMax=[]  SumI1OutMin=[]  SumI1OutMax=[]  SumI2OutMin=[]  SumI2OutMax=[]  SumI3OutMin=[]  SumI3OutMax=[]  SumDOutMin=[]  SumDOutMax=[]  SaturationOutMin=[]  SaturationOutMax=[]  IntegratorContinuousStateAttributes=''  IntegratorStateMustResolveToSignalObject=off  IntegratorRTWStateStorageClass=Auto  FilterContinuousStateAttributes=''  FilterStateMustResolveToSignalObject=off  FilterRTWStateStorageClass=Auto  DifferentiatorICPrevScaledInput=0  DifferentiatorOutMin=[]  DifferentiatorOutMax=[]
  Motores : Outport
  servos_ang_rad : Outport  Port=2
  wires:
  Radio signals/1 -> Demux/1
  Mux/1 -> Saturation/1
  Saturation/1 -> Motores/1
  Demux/1 -> Bias/1  "Throtle"
  Bias/1 -> Gain/1
  Demux/2 -> sign/1  "Yaw"
  Demux/3 -> Mux21/2  "Pitch"
  Demux/4 -> Mux21/1  "Roll"
  Mux1/1 -> Saturation1/1
  Saturation1/1 -> servos_ang_rad/1
  Sup2Servo Lin conversion/1 -> Mux1/1
  Sup2Servo Lin conversion1/1 -> Mux1/2
  Sup2Servo Lin conversion2/1 -> Mux1/3
  Ground2/1 -> Sup2Servo Lin conversion6/1
  Ground3/1 -> Sup2Servo Lin conversion5/1
  Ground4/1 -> Sup2Servo Lin conversion4/1
  Ground5/1 -> Sup2Servo Lin conversion3/1
  Sup2Servo Lin conversion3/1 -> Mux1/4
  Sup2Servo Lin conversion4/1 -> Mux1/5
  Sup2Servo Lin conversion5/1 -> Mux1/6
  Sup2Servo Lin conversion6/1 -> Mux1/7
  Sum21/1 -> roll_rate/1
  1 / rads_max/1 -> Demux13/1
  Demux13/2 -> Sum22/1
  Demux13/1 -> Sum21/1
  Sum17/1 -> yaw_rate/1
  Sum22/1 -> pitch_rate/1
  Mux13/1 -> 1 / rads_max/1
  pitch_rate/1 -> pwm_out1/2(P)
  Sum18/1 -> roll_attitude/1
  1 / rad_max/1 -> Demux10/1
  Demux10/2 -> Sum19/1
  Demux10/1 -> Sum18/1
  [rate_roll] -> Mux13/1
  Demux12/2 -> Sum19/2
  Demux12/1 -> Sum18/2
  Demux16/2 -> Sum22/2
  Demux16/1 -> Sum21/2
  roll_attitude/1 -> Mux22/1
  pitch_attitude/1 -> Mux22/2
  Demux2/3 -> 1 / rads_max_yaw/1
  [rate_pitch] -> Mux13/2
  Sum19/1 -> pitch_attitude/1
  roll_rate/1 -> pwm_out1/1(Roll)
  1 / rads_max_yaw/1 -> Sum17/1
  Mux21/1 -> Gain2/1
  Demux1/2 -> Mux15/2
  Mux15/1 -> 1 / rad_max/1
  Demux1/1 -> Mux15/1
  yaw_rate/1 -> pwm_out1/3(Y)
  Gain2/1 -> Demux12/1
  Enable/1 -> pitch_attitude/2, roll_attitude/2, yaw_rate/2, pitch_rate/2, roll_rate/2
  Mux22/1 -> Demux16/1
  Ground1/1 -> Sup2Servo Lin conversion/1
  Ground6/1 -> Sup2Servo Lin conversion1/1
  pwm_out1/4(S3) -> Saturation2/1
  pwm_out1/1(M1) -> Mux/1
  pwm_out1/2(M2) -> Mux/2
  pwm_out1/3(M3) -> Mux/3
  Saturation2/1 -> Sup2Servo Lin conversion2/1
  sign/1 -> Sum17/2
  All_meas/1 -> Bus Selector/1
  Bus Selector/1 -> Demux1/1  "<Eulr_meas_rad>"
  Bus Selector/2 -> Demux2/1  "<euler_dot_radps>"
  Demux1/3 -> Terminator/1
  Demux2/1 -> Terminator1/1
  Demux2/2 -> Terminator2/1
  Gain/1 -> pwm_out1/4(T)

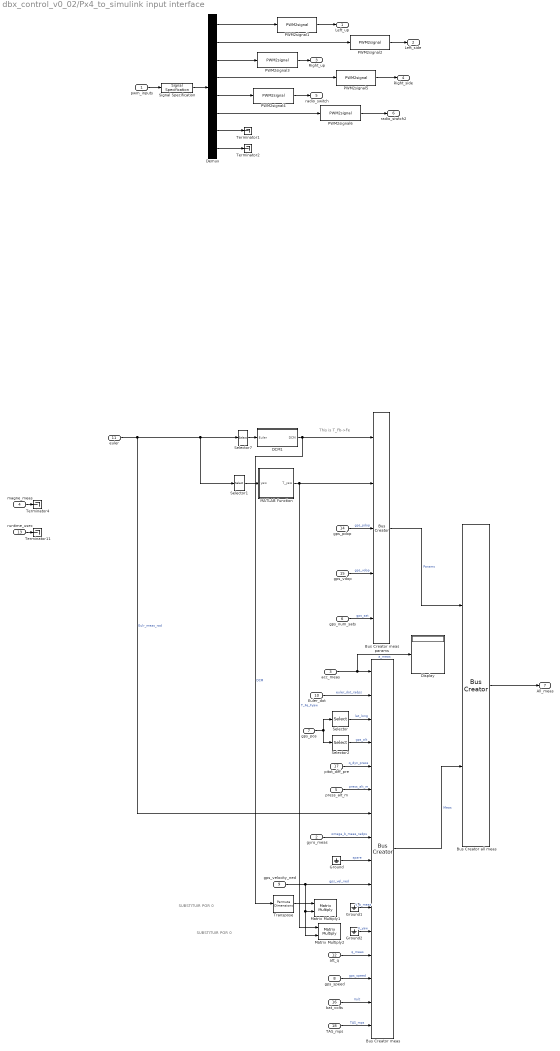
== system dbx_control_v0_02/Px4_to_simulink input interface ==
  note: SUBSTITUIR POR 0
  note: This is T_Fb->Fe
  note: SUBSTITUIR POR 0
  pwm_inputs : Inport  PortDimensions=8  SampleTime=T_ctrl
  gyro_meas : Inport  Port=2  PortDimensions=3  SampleTime=T_ctrl
  acc_meas : Inport  Port=3  PortDimensions=3  SampleTime=T_ctrl
  magne_meas : Inport  Port=4  PortDimensions=3  SampleTime=T_ctrl
  press_alt_m : Inport  Port=5  PortDimensions=1  SampleTime=T_ctrl
  gps_num_sats : Inport  Port=6  PortDimensions=1  SampleTime=T_ctrl
  gps_pos : Inport  Port=7  PortDimensions=3  SampleTime=T_ctrl
  gps_speed : Inport  Port=8  PortDimensions=1  SampleTime=T_ctrl
  gps_velocity_ned : Inport  Port=9  PortDimensions=3  SampleTime=T_ctrl
  Euler_dot : Inport  Port=10  PortDimensions=3  SampleTime=T_ctrl
  euler : Inport  Port=11  PortDimensions=3  SampleTime=T_ctrl
  att_q : Inport  Port=12  PortDimensions=4  SampleTime=T_ctrl
  runtime_usec : Inport  Port=13  PortDimensions=1  SampleTime=T_ctrl
  gps_pdop : Inport  Port=14  PortDimensions=1  SampleTime=T_ctrl
  gps_vdop : Inport  Port=15  PortDimensions=1  SampleTime=T_ctrl
  bat_volts : Inport  Port=16  PortDimensions=1  SampleTime=T_ctrl
  pitot_diff_pre : Inport  Port=17  SampleTime=T_ctrl
  TAS_mps : Inport  Port=18  SampleTime=T_ctrl
  Bus Creator all meas : BusCreator  Inputs=2
  Bus Creator meas : BusCreator  Inputs=16
  Bus Creator meas params : BusCreator  Inputs=5
  DCM1 : Subsystem  TreatAsAtomicUnit=on
  Demux : Demux  Outputs=8
  Display : Display
  Ground : Ground
  Ground1 : Ground
  Ground2 : Ground
  MATLAB Function : MATLAB Function  TreatAsAtomicUnit=on
  Matrix Multiply1 : Product  Multiplication=Matrix(*)
  Matrix Multiply2 : Product  Multiplication=Matrix(*)
  PWM2signal{1..6} (6 alike) : DBX_model/PWM2signal  c=2000  a=1000  d=1  b=-1
  Selector : Selector  InputPortWidth=3  Indices=[1,2]
  Selector1 : Selector  InputPortWidth=3  Indices=3
  Selector2 : Selector  InputPortWidth=3  Indices=3
  Selector7 : Selector  InputPortWidth=3  Indices=[3 2 1]
  Signal Specification : SignalSpecification  Dimensions=8
  Terminator{1..2,4,11} (4 alike) : Terminator
  Transpose : PermuteDimensions
  Left_up : Outport
  Left_side : Outport  Port=2
  Right_up : Outport  Port=3
  Right_side : Outport  Port=4
  radio_switch : Outport  Port=5
  radio_siwtch2 : Outport  Port=6
  All_meas : Outport  Port=7
  wires:
  PWM2signal1/1 -> Left_up/1
  PWM2signal2/1 -> Left_side/1
  PWM2signal3/1 -> Right_up/1
  PWM2signal5/1 -> Right_side/1
  Bus Creator all meas/1 -> All_meas/1
  PWM2signal4/1 -> radio_switch/1
  att_q/1 -> Bus Creator meas/13  "q_meas"
  euler/1 -> Bus Creator meas/7, Selector1/1, Selector7/1  "Eulr_meas_rad"
  Euler_dot/1 -> Bus Creator meas/2  "euler_dot_radps"
  bat_volts/1 -> Bus Creator meas/15  "Volt"
  Bus Creator meas/1 -> Bus Creator all meas/2  "Meas"
  Bus Creator meas params/1 -> Bus Creator all meas/1  "Params"
  DCM1/1(DCM) -> Transpose/1, Bus Creator meas params/1  "DCM"
  acc_meas/1 -> Display/1, Bus Creator meas/1  "a_meas"
  gps_pdop/1 -> Bus Creator meas params/3  "gps_pdop"
  gps_num_sats/1 -> Bus Creator meas params/5  "gps_sat"
  gps_vdop/1 -> Bus Creator meas params/4  "gps_vdop"
  Selector7/1 -> DCM1/1(Euler)
  Selector1/1 -> MATLAB Function/1(yaw)
  MATLAB Function/1(T_yaw) -> Matrix Multiply2/1, Bus Creator meas params/2  "T_Fe_Fyaw"
  Demux/1 -> PWM2signal1/1
  Demux/2 -> PWM2signal2/1
  Demux/3 -> PWM2signal3/1
  Demux/4 -> PWM2signal5/1
  Demux/5 -> PWM2signal4/1
  pwm_inputs/1 -> Signal Specification/1
  Demux/6 -> PWM2signal6/1
  Demux/7 -> Terminator1/1
  Demux/8 -> Terminator2/1
  gyro_meas/1 -> Bus Creator meas/8  "omega_b_meas_radps"
  magne_meas/1 -> Terminator4/1
  press_alt_m/1 -> Bus Creator meas/6  "press_alt_m"
  gps_pos/1 -> Selector2/1, Selector/1
  gps_speed/1 -> Bus Creator meas/14  "gps_speed"
  gps_velocity_ned/1 -> Bus Creator meas/10, Matrix Multiply2/2, Matrix Multiply1/2  "gps_vel_ned"
  runtime_usec/1 -> Terminator11/1
  Signal Specification/1 -> Demux/1
  PWM2signal6/1 -> radio_siwtch2/1
  pitot_diff_pre/1 -> Bus Creator meas/5  "q_dyn_press"
  Selector/1 -> Bus Creator meas/3  "lat_long"
  Selector2/1 -> Bus Creator meas/4  "gps_alt"
  TAS_mps/1 -> Bus Creator meas/16  "TAS_mps"
  Transpose/1 -> Matrix Multiply1/1
  Ground1/1 -> Bus Creator meas/11  "V_b_meas"
  Ground2/1 -> Bus Creator meas/12  "V_yaw"
  Ground/1 -> Bus Creator meas/9  "spare"

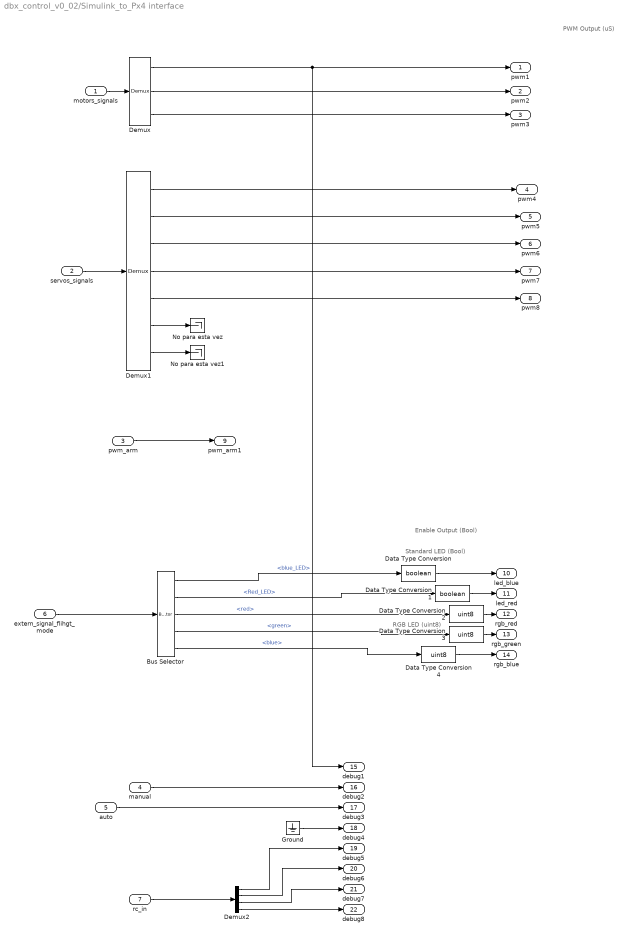
== system dbx_control_v0_02/Simulink_to_Px4 interface ==
  note: RGB LED (uint8)
  note: Standard LED (Bool)
  note: PWM Output (uS)
  note: Enable Output (Bool)
  motors_signals : Inport
  servos_signals : Inport  Port=2
  pwm_arm : Inport  Port=3
  manual : Inport  Port=4
  auto : Inport  Port=5
  extern_signal_flihgt_mode : Inport  Port=6
  rc_in : Inport  Port=7
  Bus Selector : BusSelector  OutputSignals=blue_LED,Red_LED,RGBLED.red,RGBLED.green,RGBLED.blue
  Data Type Conversion : DataTypeConversion  OutDataTypeStr=boolean
  Data Type Conversion1 : DataTypeConversion  OutDataTypeStr=boolean
  Data Type Conversion2 : DataTypeConversion  OutDataTypeStr=uint8
  Data Type Conversion3 : DataTypeConversion  OutDataTypeStr=uint8
  Data Type Conversion4 : DataTypeConversion  OutDataTypeStr=uint8
  Demux : Demux  Outputs=3
  Demux1 : Demux  Outputs=7
  Demux2 : Demux
  Ground : Ground
  No para esta vez : Terminator
  No para esta vez1 : Terminator
  pwm1 : Outport  PortDimensions=1  SampleTime=T_ctrl
  pwm2 : Outport  Port=2  PortDimensions=1  SampleTime=T_ctrl
  pwm3 : Outport  Port=3  PortDimensions=1  SampleTime=T_ctrl
  pwm4 : Outport  Port=4  PortDimensions=1  SampleTime=T_ctrl
  pwm5 : Outport  Port=5  PortDimensions=1  SampleTime=T_ctrl
  pwm6 : Outport  Port=6  PortDimensions=1  SampleTime=T_ctrl
  pwm7 : Outport  Port=7  PortDimensions=1  SampleTime=T_ctrl
  pwm8 : Outport  Port=8  PortDimensions=1  SampleTime=T_ctrl
  pwm_arm1 : Outport  Port=9  PortDimensions=1  SampleTime=T_ctrl
  led_blue : Outport  Port=10  OutDataTypeStr=boolean  PortDimensions=1  SampleTime=T_ctrl
  led_red : Outport  Port=11  OutDataTypeStr=boolean  PortDimensions=1  SampleTime=T_ctrl
  rgb_red : Outport  Port=12  OutDataTypeStr=uint8  PortDimensions=1  SampleTime=T_ctrl
  rgb_green : Outport  Port=13  OutDataTypeStr=uint8  PortDimensions=1  SampleTime=T_ctrl
  rgb_blue : Outport  Port=14  OutDataTypeStr=uint8  PortDimensions=1  SampleTime=T_ctrl
  debug1 : Outport  Port=15  PortDimensions=1  SampleTime=T_ctrl
  debug2 : Outport  Port=16  PortDimensions=1  SampleTime=T_ctrl
  debug3 : Outport  Port=17  PortDimensions=1  SampleTime=T_ctrl
  debug4 : Outport  Port=18  PortDimensions=1  SampleTime=T_ctrl
  debug5 : Outport  Port=19  PortDimensions=1  SampleTime=T_ctrl
  debug6 : Outport  Port=20  PortDimensions=1  SampleTime=T_ctrl
  debug7 : Outport  Port=21  PortDimensions=1  SampleTime=T_ctrl
  debug8 : Outport  Port=22  PortDimensions=1  SampleTime=T_ctrl
  wires:
  extern_signal_flihgt_mode/1 -> Bus Selector/1
  Bus Selector/2 -> Data Type Conversion1/1  "<Red_LED>"
  pwm_arm/1 -> pwm_arm1/1
  Bus Selector/3 -> Data Type Conversion2/1  "<red>"
  Bus Selector/4 -> Data Type Conversion3/1  "<green>"
  Bus Selector/5 -> Data Type Conversion4/1  "<blue>"
  Data Type Conversion/1 -> led_blue/1
  Data Type Conversion1/1 -> led_red/1
  Data Type Conversion2/1 -> rgb_red/1
  Data Type Conversion3/1 -> rgb_green/1
  Data Type Conversion4/1 -> rgb_blue/1
  Bus Selector/1 -> Data Type Conversion/1  "<blue_LED>"
  motors_signals/1 -> Demux/1
  Demux/1 -> debug1/1, pwm1/1
  Demux/2 -> pwm2/1
  servos_signals/1 -> Demux1/1
  rc_in/1 -> Demux2/1
  manual/1 -> debug2/1
  auto/1 -> debug3/1
  Demux2/4 -> debug8/1
  Demux2/3 -> debug7/1
  Demux2/2 -> debug6/1
  Demux2/1 -> debug5/1
  Ground/1 -> debug4/1
  Demux/3 -> pwm3/1
  Demux1/1 -> pwm4/1
  Demux1/2 -> pwm5/1
  Demux1/3 -> pwm6/1
  Demux1/4 -> pwm7/1
  Demux1/5 -> pwm8/1
  Demux1/6 -> No para esta vez/1
  Demux1/7 -> No para esta vez1/1

== system dbx_control_v0_02/Status signals ==
  manual : Inport
  auto : Inport  Port=2
  pwm_arm : Inport  Port=3
  Ground1 : Ground
  Logical Operator1 : Logic  Operator=NOT  IconShape=distinctive  AllPortsSameDT=off  OutDataTypeStr=boolean
  Beep : Outport
  Red_LED : Outport  Port=2
  blue_LED : Outport  Port=3
  blue_RGBLED : Outport  Port=4
  Red_RGBLED : Outport  Port=5
  green_RGBLED : Outport  Port=6
  wires:
  Ground1/1 -> Beep/1
  manual/1 -> Red_RGBLED/1, Red_LED/1
  auto/1 -> blue_RGBLED/1, blue_LED/1
  pwm_arm/1 -> Logical Operator1/1
  Logical Operator1/1 -> green_RGBLED/1

== system dbx_control_v0_02/Auto-mode autopiloto/Activation bus ==
  Activation1 : Inport
  Activation : Inport  Port=2
  Bus Creator : BusCreator  Inputs=6
  Ground{,1..3} (4 alike) : Ground
  Activation bus : Outport
  wires:
  Ground1/1 -> Bus Creator/2  "alt_act"
  Ground2/1 -> Bus Creator/3  "vel_yaw_xy_act"
  Ground3/1 -> Bus Creator/4  "vel_yaw_z_act"
  Activation1/1 -> Bus Creator/5  "euler_act"
  Activation/1 -> Bus Creator/6  "b_rates_act"
  Bus Creator/1 -> Activation bus/1
  Ground/1 -> Bus Creator/1  "pos_xy_act"

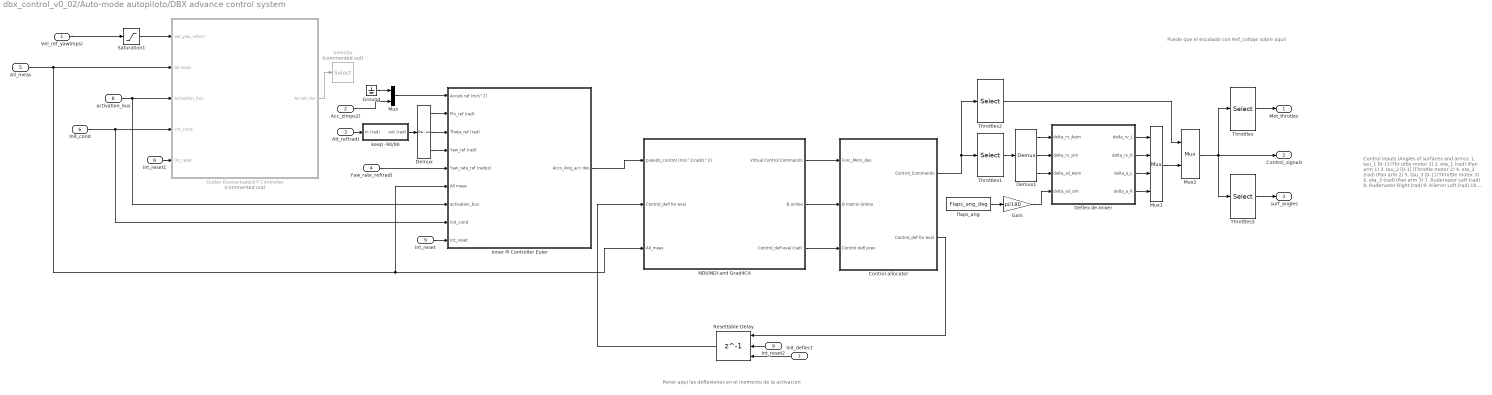
== system dbx_control_v0_02/Auto-mode autopiloto/DBX advance control system ==
  note: Puede que el escalado con Ref_coltaje sobre aqui!
  note: Poner aqui las deflexiones en el momento de la activacion
  note: Control inputs (Angles  of surfaces and arms):
      |
      | 1. tau_1 [0-1] (Thr ottle motor 1)
      | 2. eta_1 (rad)  (Pan arm 1)
      |
      | 3. tau_2 [0-1] (Throttle motor 2)
      | 4. eta_2 (rad)  (Pan arm 2)
      |
      | 5. tau_3 [0-1] (Throttle motor 3)
      | 6. eta_3 (rad)  (Pan arm  3)
      |
      | 7. Rudervator Left (rad)
      | 8. Rudervator Right (rad)
      | 9. Aileron Left (rad)
      | 10. Aielron Right (rad)
  Vel_ref_yaw(mps) : Inport
  Acc_z(mps2) : Inport  Port=2
  Att_ref(rad) : Inport  Port=3
  Yaw_rate_ref(rad) : Inport  Port=4
  All_meas : Inport  Port=5
  Init_cond : Inport  Port=6
  Init_deflect : Inport  Port=7  PortDimensions=[9,1]
  activation_bus : Inport  Port=8
  Int_reset : Inport  Port=9
  Control allocator : Subsystem  RTWFcnName=abc  RTWFileName=asas  VariantControl=Control Allocator: NO RECONFIG
      settings: MinAlgLoopOccurrences=on  RTWFcnNameOpts=User specified  RTWFileNameOpts=User specified
  Deflex de-mixer : Subsystem  TreatAsAtomicUnit=on
  Demux : Demux  Outputs=3
  Demux1 : Demux  Outputs=3
  Gain : Gain  Gain=pi/180
  Ground : Ground
  Inner PI Controller Euler : Subsystem  VariantControl=PI_quat
  Int_reset1 : InportShadow  Port=9
  Int_reset2 : InportShadow  Port=9
  Mux : Mux  Inputs=[2,1]
  Mux1 : Mux
  Mux2 : Mux  Inputs=[6,4]
  NDI/INDI and Grad4CA : Subsystem  Variant=on  VariantControl=NDI: NO RECONFIG  OverrideUsingVariant=NDI_incremental_grad
  Outter Overactuated P Controller : Subsystem  Commented=on  VariantControl=Overactuated P Controller
  Resettable Delay : Delay  DelayLength=1  InitialConditionSource=Input port  ExternalReset=Either  InputProcessing=Inherited  SampleTime=T_ctrl
      settings: InputPortMap=u0,r5,p4
  Saturation1 : Saturate  UpperLimit=[10,10,v_i0]'  LowerLimit=-[10,10,2*v_i0]'
  Selector : Selector  Commented=on  InputPortWidth=3  Indices=1:2
  Throttles : Selector  InputPortWidth=10  Indices=[1,3,5]
  Throttles1 : Selector  InputPortWidth=9  Indices=[7:9]
  Throttles2 : Selector  InputPortWidth=9  Indices=[1:6]
  Throttles3 : Selector  InputPortWidth=10  Indices=[2,4,6,7,8,9,10]
  flaps_ang : Constant  Value=Flaps_ang_deg
  keep -90/90 : Subsystem
  Mot_throtles : Outport
  Control_signals : Outport  Port=2
  surf_angles : Outport  Port=3
  wires:
  All_meas/1 -> Inner PI Controller Euler/6(All meas), NDI/INDI and Grad4CA/3(All_meas), Outter Overactuated P Controller/2(All meas)
  NDI/INDI and Grad4CA/3(Control_defl eval (rad)) -> Control allocator/3(Control defl prev)
  keep -90/90/1(out (rad)) -> Demux/1
  Demux/3 -> Inner PI Controller Euler/4(Yaw_ref (rad))
  Demux/2 -> Inner PI Controller Euler/3(Theta_ref (rad))
  Demux/1 -> Inner PI Controller Euler/2(Phi_ref (rad))
  Att_ref(rad)/1 -> keep -90/90/1(in (rad))
  Throttles/1 -> Mot_throtles/1
  Control allocator/1(Control_Commands) -> Throttles2/1, Throttles1/1
  Resettable Delay/1 -> NDI/INDI and Grad4CA/2(Control_defl for eval)
  Vel_ref_yaw(mps)/1 -> Saturation1/1
  Saturation1/1 -> Outter Overactuated P Controller/1(Vel_yaw_ref(m))
  Init_cond/1 -> Inner PI Controller Euler/8(init_cond), Outter Overactuated P Controller/4(init_cond)
  activation_bus/1 -> Inner PI Controller Euler/7(activation_bus), Outter Overactuated P Controller/3(activation_bus)
  Control allocator/2(Control_def for eval) -> Resettable Delay/1
  NDI/INDI and Grad4CA/2(B online) -> Control allocator/2(B matrix Online)
  Inner PI Controller Euler/1(Accs_Ang_acc des) -> NDI/INDI and Grad4CA/1(pseudo_control (m/s^2;rad/s^2))
  Demux1/2 -> Deflex de-mixer/2(delta_rv_sim)
  Demux1/3 -> Deflex de-mixer/3(delta_ail_Asim)
  Demux1/1 -> Deflex de-mixer/1(delta_rv_Asim)
  Throttles1/1 -> Demux1/1
  Throttles2/1 -> Mux2/1
  Deflex de-mixer/1(delta_rv_L) -> Mux1/1
  Deflex de-mixer/2(delta_rv_R) -> Mux1/2
  Deflex de-mixer/3(delta_a_L) -> Mux1/3
  Deflex de-mixer/4(delta_a_R) -> Mux1/4
  Mux1/1 -> Mux2/2
  Mux2/1 -> Throttles3/1, Throttles/1, Control_signals/1
  Throttles3/1 -> surf_angles/1
  Yaw_rate_ref(rad)/1 -> Inner PI Controller Euler/5(Yaw_rate_ref (radps))
  Int_reset/1 -> Inner PI Controller Euler/9(Int_reset)
  Int_reset1/1 -> Outter Overactuated P Controller/5(Int_reset)
  Acc_z(mps2)/1 -> Mux/2
  Mux/1 -> Inner PI Controller Euler/1(Accels ref (m/s^2))
  Init_deflect/1 -> Resettable Delay/3
  Int_reset2/1 -> Resettable Delay/2
  NDI/INDI and Grad4CA/1(Virtual Control Commands) -> Control allocator/1(Forc_Mom_des)
  Outter Overactuated P Controller/1(Accels des) -> Selector/1
  Ground/1 -> Mux/1
  flaps_ang/1 -> Gain/1
  Gain/1 -> Deflex de-mixer/4(delta_ail_sim)

== system dbx_control_v0_02/Auto-mode autopiloto/Initial conditions ==
  All_meas : Inport
  Bus Creator1 : BusCreator  Inputs=6
  Bus Selector : BusSelector  OutputSignals=Meas.Eulr_meas_rad,Meas.omega_b_meas_radps
  Ground{,1..3} (4 alike) : Ground
  Init_cond : Outport
  wires:
  Ground2/1 -> Bus Creator1/3  "vel_yaw_xy_init"
  Bus Selector/2 -> Bus Creator1/6  "<omega_b_meas_radps>"
  Ground3/1 -> Bus Creator1/4  "vel_yaw_z_init"
  Bus Selector/1 -> Bus Creator1/5  "<Eulr_meas_rad>"
  Ground/1 -> Bus Creator1/1  "pos_xy_init"
  Ground1/1 -> Bus Creator1/2  "alt_init"
  All_meas/1 -> Bus Selector/1
  Bus Creator1/1 -> Init_cond/1

== system dbx_control_v0_02/Auto-mode autopiloto/Sensibilidades Radio ==
  Radio_in : Inport
  Demux : Demux
  Demux1 : Demux  Outputs=2
  Divide : Product  Inputs=**
  Divide1 : Product  Inputs=**
  Gain : Gain  Gain=-Throtle_sens
  Mux : Mux  Inputs=2
  Saturation : Saturate  UpperLimit=9  LowerLimit=-5
  Yaw_sens : Constant  Value=Yaw_sens
  deg2rad : Gain  Gain=pi/180
  deg2rad1 : Gain  Gain=pi/180
  deg2rad2 : Gain  Gain=[1,-1]
  roll_pich_sens : Constant  Value=Roll_pich_sens
  Acc_z_mps2 : Outport
  Yaw(radps) : Outport  Port=2
  Pitch(rad) : Outport  Port=3
  Roll(rad) : Outport  Port=4
  wires:
  Demux/1 -> Gain/1  "Throtle"
  Demux/2 -> Divide/1  "Yaw"
  Demux/3 -> Mux/2  "Pitch"
  Demux/4 -> Mux/1  "Roll"
  Radio_in/1 -> Demux/1
  Divide/1 -> Yaw(radps)/1
  Mux/1 -> Divide1/1
  Divide1/1 -> Demux1/1
  Demux1/1 -> Roll(rad)/1
  Demux1/2 -> Pitch(rad)/1
  Gain/1 -> Saturation/1
  Saturation/1 -> Acc_z_mps2/1
  Yaw_sens/1 -> deg2rad/1
  deg2rad/1 -> Divide/2
  roll_pich_sens/1 -> deg2rad1/1
  deg2rad1/1 -> deg2rad2/1
  deg2rad2/1 -> Divide1/2

== system dbx_control_v0_02/Px4_to_simulink input interface/DCM1 ==
  Euler : Inport  PortDimensions=3
  Fcn11 : Fcn  Expr=u(5)*u(4)
  Fcn12 : Fcn  Expr=u(5)*u(1)
  Fcn13 : Fcn  Expr=-u(2)
  Fcn21 : Fcn  Expr=u(3)*u(2)*u(4) - u(6)*u(1)
  Fcn22 : Fcn  Expr=u(3)*u(2)*u(1) + u(6)*u(4)
  Fcn23 : Fcn  Expr=u(3)*u(5)
  Fcn31 : Fcn  Expr=u(6)*u(2)*u(4) + u(3)*u(1)
  Fcn32 : Fcn  Expr=u(6)*u(2)*u(1) - u(3)*u(4)
  Fcn33 : Fcn  Expr=u(6)*u(5)
  Mux : Mux  Inputs=2
  Mux1 : Mux  Inputs=9
  Reshape : Reshape  OutputDimensionality=Customize  OutputDimensions=[3,3]
  sincos : Trigonometry  Operator=sincos
  DCM : Outport  PortDimensions=[3,3]
  wires:
  Fcn33/1 -> Mux1/9
  Fcn32/1 -> Mux1/8
  Fcn23/1 -> Mux1/6
  Fcn22/1 -> Mux1/5
  Fcn31/1 -> Mux1/7
  Fcn21/1 -> Mux1/4
  Fcn13/1 -> Mux1/3
  Fcn12/1 -> Mux1/2
  Fcn11/1 -> Mux1/1
  Mux/1 -> Fcn22/1, Fcn23/1, Fcn31/1, Fcn33/1, Fcn32/1, Fcn21/1, Fcn13/1, Fcn12/1, Fcn11/1
  sincos/2 -> Mux/2
  sincos/1 -> Mux/1
  Reshape/1 -> DCM/1
  Euler/1 -> sincos/1
  Mux1/1 -> Reshape/1
